simulink library "TestSeq_slave_lib"  (Simulink 8.1)
settings: Solver=ode45  StartTime=0.0  StopTime=10.0  RelTol=1e-3
undefined symbols (not defined in the file): DiscIntNeverNeededParam, Ts
libraries: simulink x24, simulink_extras x1
settings Model: Creator=ch24070  LastModifiedBy=pkoralew

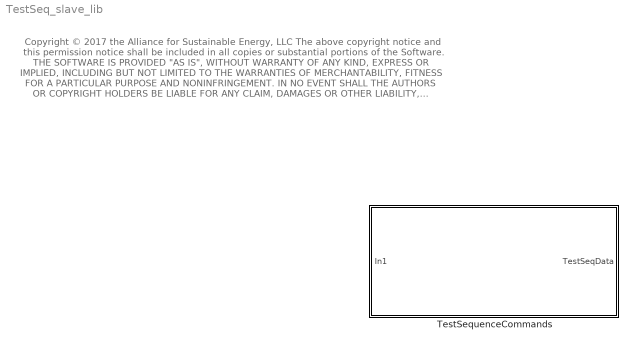
== system TestSeq_slave_lib ==
  note: Copyright © 2017 the Alliance for Sustainable Energy, LLC
      |
      | The above copyright notice and this permission notice shall be included in all copies or substantial portions of the Software.
      |
      | THE SOFTWARE IS PROVIDED "AS IS", WITHOUT WARRANTY OF ANY KIND, EXPRESS OR IMPLIED, INCLUDING
      | BUT NOT LIMITED TO THE WARRANTIES OF MERCHANTABILITY, FITNESS FOR A PARTICULAR PURPOSE AND
      | NONINFRINGEMENT. IN NO EVENT SHALL THE AUTHORS OR COPYRIGHT HOLDERS BE LIABLE FOR ANY CLAIM,
      |  DAMAGES OR OTHER LIABILITY, WHETHER IN AN ACTION OF CONTRACT, TORT OR OTHERWISE, ARISING FROM,
      | OUT OF OR IN CONNECTION WITH THE SOFTWARE OR THE USE OR OTHER DEALINGS IN THE SOFTWARE
  TestSequenceCommands : Subsystem

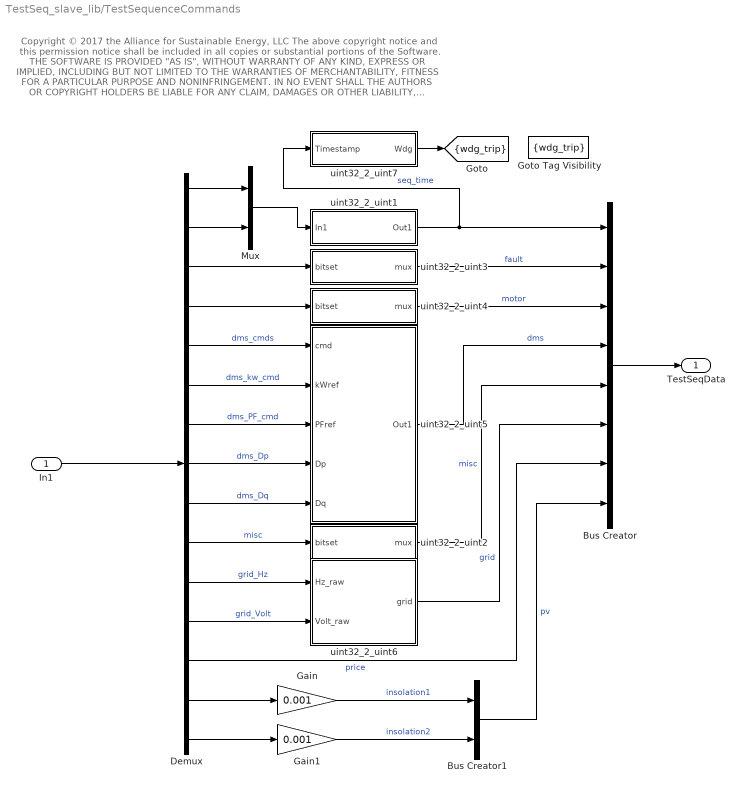
== system TestSeq_slave_lib/TestSequenceCommands ==
  note: Copyright © 2017 the Alliance for Sustainable Energy, LLC
      |
      | The above copyright notice and this permission notice shall be included in all copies or substantial portions of the Software.
      |
      | THE SOFTWARE IS PROVIDED "AS IS", WITHOUT WARRANTY OF ANY KIND, EXPRESS OR IMPLIED, INCLUDING
      | BUT NOT LIMITED TO THE WARRANTIES OF MERCHANTABILITY, FITNESS FOR A PARTICULAR PURPOSE AND
      | NONINFRINGEMENT. IN NO EVENT SHALL THE AUTHORS OR COPYRIGHT HOLDERS BE LIABLE FOR ANY CLAIM,
      |  DAMAGES OR OTHER LIABILITY, WHETHER IN AN ACTION OF CONTRACT, TORT OR OTHERWISE, ARISING FROM,
      | OUT OF OR IN CONNECTION WITH THE SOFTWARE OR THE USE OR OTHER DEALINGS IN THE SOFTWARE
  In1 : Inport
  Bus Creator : BusCreator  Inputs=8
  Bus Creator1 : BusCreator  Inputs=2
  Demux : Demux  Outputs=15
  Gain : Gain  Gain=0.001
  Gain1 : Gain  Gain=0.001
  Goto Tag Visibility : GotoTagVisibility  GotoTag=wdg_trip
  Mux : Mux  Inputs=2
  uint32_2_uint1 : Subsystem
      mask Display: disp('uint16_2_uint32');
  uint32_2_uint2 : Subsystem
  uint32_2_uint3 : Subsystem
  uint32_2_uint4 : Subsystem
  uint32_2_uint5 : Subsystem
  uint32_2_uint6 : Subsystem
  uint32_2_uint7 : Subsystem
      mask Display: disp('Watchdog\nT=2s');
  TestSeqData : Outport
  tag scope: wdg_trip=scoped
  wires:
  Gain1/1 -> Bus Creator1/2  "insolation2"
  Gain/1 -> Bus Creator1/1  "insolation1"
  Bus Creator1/1 -> Bus Creator/8  "pv"
  Demux/15 -> Gain1/1
  Demux/14 -> Gain/1
  uint32_2_uint6/1(grid) -> Bus Creator/6  "grid"
  uint32_2_uint7/1(Wdg) -> [wdg_trip]
  Demux/13 -> Bus Creator/7  "price"
  uint32_2_uint2/1(mux) -> Bus Creator/5  "misc"
  uint32_2_uint5/1(Out1) -> Bus Creator/4  "dms"
  uint32_2_uint4/1(mux) -> Bus Creator/3  "motor"
  uint32_2_uint3/1(mux) -> Bus Creator/2  "fault"
  Mux/1 -> uint32_2_uint1/1(In1)
  Demux/2 -> Mux/2
  Demux/1 -> Mux/1
  Demux/12 -> uint32_2_uint6/2(Volt_raw)  "grid_Volt"
  Demux/3 -> uint32_2_uint3/1(bitset)
  Demux/4 -> uint32_2_uint4/1(bitset)
  Demux/5 -> uint32_2_uint5/1(cmd)  "dms_cmds"
  Demux/6 -> uint32_2_uint5/2(kWref)  "dms_kw_cmd"
  Demux/7 -> uint32_2_uint5/3(PFref)  "dms_PF_cmd"
  Demux/8 -> uint32_2_uint5/4(Dp)  "dms_Dp"
  Demux/9 -> uint32_2_uint5/5(Dq)  "dms_Dq"
  Demux/10 -> uint32_2_uint2/1(bitset)  "misc"
  uint32_2_uint1/1(Out1) -> Bus Creator/1, uint32_2_uint7/1(Timestamp)  "seq_time"
  In1/1 -> Demux/1
  Demux/11 -> uint32_2_uint6/1(Hz_raw)  "grid_Hz"
  Bus Creator/1 -> TestSeqData/1

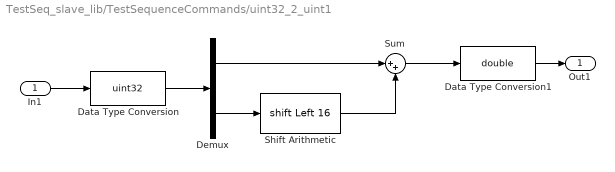
== system TestSeq_slave_lib/TestSequenceCommands/uint32_2_uint1 ==
  In1 : Inport
  Data Type Conversion : DataTypeConversion  OutDataTypeStr=uint32
  Data Type Conversion1 : DataTypeConversion  OutDataTypeStr=double
  Demux : Demux  Outputs=2
  Shift Arithmetic : ArithShift  BitShiftNumber=16  BitShiftDirection=Left
  Sum : Sum  Inputs=|++
  Out1 : Outport
  wires:
  Data Type Conversion/1 -> Demux/1
  Demux/1 -> Sum/1
  Demux/2 -> Shift Arithmetic/1
  Data Type Conversion1/1 -> Out1/1
  In1/1 -> Data Type Conversion/1
  Sum/1 -> Data Type Conversion1/1
  Shift Arithmetic/1 -> Sum/2

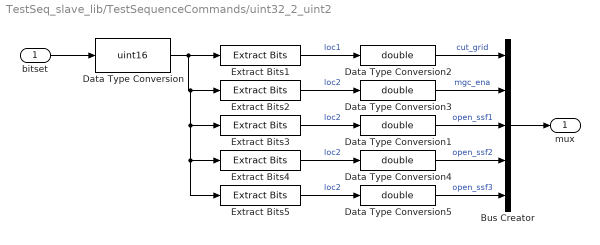
== system TestSeq_slave_lib/TestSequenceCommands/uint32_2_uint2 ==
  bitset : Inport
  Bus Creator : BusCreator  Inputs=5
  Data Type Conversion : DataTypeConversion  OutDataTypeStr=uint16
  Data Type Conversion{1..5} (5 alike) : DataTypeConversion  OutDataTypeStr=double
  Extract Bits1 : simulink/Logic and Bit Operations/Extract Bits  bitsToExtract=Range of bits  numBits=8  bitIdxRange=[0]  outScalingMode=Treat bit field as an integer
  Extract Bits2 : simulink/Logic and Bit Operations/Extract Bits  bitsToExtract=Range of bits  numBits=8  bitIdxRange=1  outScalingMode=Treat bit field as an integer
  Extract Bits3 : simulink/Logic and Bit Operations/Extract Bits  bitsToExtract=Range of bits  numBits=8  bitIdxRange=2  outScalingMode=Treat bit field as an integer
  Extract Bits4 : simulink/Logic and Bit Operations/Extract Bits  bitsToExtract=Range of bits  numBits=8  bitIdxRange=3  outScalingMode=Treat bit field as an integer
  Extract Bits5 : simulink/Logic and Bit Operations/Extract Bits  bitsToExtract=Range of bits  numBits=8  bitIdxRange=4  outScalingMode=Treat bit field as an integer
  mux : Outport
  wires:
  Extract Bits5/1 -> Data Type Conversion5/1  "loc2"
  Data Type Conversion5/1 -> Bus Creator/5  "open_ssf3"
  Extract Bits4/1 -> Data Type Conversion4/1  "loc2"
  Data Type Conversion4/1 -> Bus Creator/4  "open_ssf2"
  Data Type Conversion/1 -> Extract Bits1/1, Extract Bits2/1, Extract Bits3/1, Extract Bits4/1, Extract Bits5/1
  Extract Bits3/1 -> Data Type Conversion1/1  "loc2"
  Data Type Conversion1/1 -> Bus Creator/3  "open_ssf1"
  Extract Bits2/1 -> Data Type Conversion3/1  "loc2"
  Extract Bits1/1 -> Data Type Conversion2/1  "loc1"
  bitset/1 -> Data Type Conversion/1
  Bus Creator/1 -> mux/1
  Data Type Conversion2/1 -> Bus Creator/1  "cut_grid"
  Data Type Conversion3/1 -> Bus Creator/2  "mgc_ena"

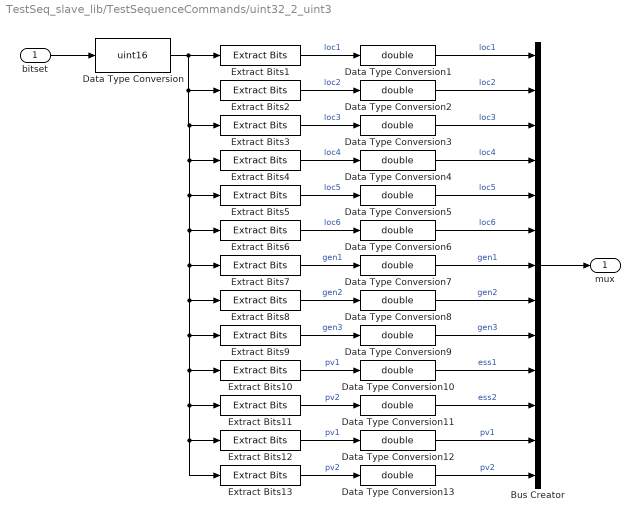
== system TestSeq_slave_lib/TestSequenceCommands/uint32_2_uint3 ==
  bitset : Inport
  Bus Creator : BusCreator  Inputs=13
  Data Type Conversion : DataTypeConversion  OutDataTypeStr=uint16
  Data Type Conversion{1..13} (13 alike) : DataTypeConversion  OutDataTypeStr=double
  Extract Bits1 : simulink/Logic and Bit Operations/Extract Bits  bitsToExtract=Range of bits  numBits=8  bitIdxRange=[0]  outScalingMode=Treat bit field as an integer
  Extract Bits10 : simulink/Logic and Bit Operations/Extract Bits  bitsToExtract=Range of bits  numBits=8  bitIdxRange=9  outScalingMode=Treat bit field as an integer
  Extract Bits11 : simulink/Logic and Bit Operations/Extract Bits  bitsToExtract=Range of bits  numBits=8  bitIdxRange=10  outScalingMode=Treat bit field as an integer
  Extract Bits12 : simulink/Logic and Bit Operations/Extract Bits  bitsToExtract=Range of bits  numBits=8  bitIdxRange=11  outScalingMode=Treat bit field as an integer
  Extract Bits13 : simulink/Logic and Bit Operations/Extract Bits  bitsToExtract=Range of bits  numBits=8  bitIdxRange=12  outScalingMode=Treat bit field as an integer
  Extract Bits2 : simulink/Logic and Bit Operations/Extract Bits  bitsToExtract=Range of bits  numBits=8  bitIdxRange=1  outScalingMode=Treat bit field as an integer
  Extract Bits3 : simulink/Logic and Bit Operations/Extract Bits  bitsToExtract=Range of bits  numBits=8  bitIdxRange=2  outScalingMode=Treat bit field as an integer
  Extract Bits4 : simulink/Logic and Bit Operations/Extract Bits  bitsToExtract=Range of bits  numBits=8  bitIdxRange=3  outScalingMode=Treat bit field as an integer
  Extract Bits5 : simulink/Logic and Bit Operations/Extract Bits  bitsToExtract=Range of bits  numBits=8  bitIdxRange=4  outScalingMode=Treat bit field as an integer
  Extract Bits6 : simulink/Logic and Bit Operations/Extract Bits  bitsToExtract=Range of bits  numBits=8  bitIdxRange=5  outScalingMode=Treat bit field as an integer
  Extract Bits7 : simulink/Logic and Bit Operations/Extract Bits  bitsToExtract=Range of bits  numBits=8  bitIdxRange=6  outScalingMode=Treat bit field as an integer
  Extract Bits8 : simulink/Logic and Bit Operations/Extract Bits  bitsToExtract=Range of bits  numBits=8  bitIdxRange=7  outScalingMode=Treat bit field as an integer
  Extract Bits9 : simulink/Logic and Bit Operations/Extract Bits  bitsToExtract=Range of bits  numBits=8  bitIdxRange=8  outScalingMode=Treat bit field as an integer
  mux : Outport
  wires:
  Extract Bits13/1 -> Data Type Conversion13/1  "pv2"
  Extract Bits12/1 -> Data Type Conversion12/1  "pv1"
  Data Type Conversion13/1 -> Bus Creator/13  "pv2"
  Data Type Conversion12/1 -> Bus Creator/12  "pv1"
  Data Type Conversion/1 -> Extract Bits2/1, Extract Bits3/1, Extract Bits13/1, Extract Bits12/1, Extract Bits11/1, Extract Bits10/1, Extract Bits9/1, Extract Bits8/1, Extract Bits7/1, Extract Bits6/1, Extract Bits5/1, Extract Bits4/1, Extract Bits1/1
  Extract Bits11/1 -> Data Type Conversion11/1  "pv2"
  Extract Bits10/1 -> Data Type Conversion10/1  "pv1"
  Extract Bits9/1 -> Data Type Conversion9/1  "gen3"
  Extract Bits8/1 -> Data Type Conversion8/1  "gen2"
  Extract Bits7/1 -> Data Type Conversion7/1  "gen1"
  Extract Bits6/1 -> Data Type Conversion6/1  "loc6"
  Extract Bits5/1 -> Data Type Conversion5/1  "loc5"
  Extract Bits4/1 -> Data Type Conversion4/1  "loc4"
  Extract Bits3/1 -> Data Type Conversion3/1  "loc3"
  Extract Bits2/1 -> Data Type Conversion2/1  "loc2"
  Extract Bits1/1 -> Data Type Conversion1/1  "loc1"
  Data Type Conversion11/1 -> Bus Creator/11  "ess2"
  Data Type Conversion10/1 -> Bus Creator/10  "ess1"
  Data Type Conversion9/1 -> Bus Creator/9  "gen3"
  Data Type Conversion8/1 -> Bus Creator/8  "gen2"
  Data Type Conversion7/1 -> Bus Creator/7  "gen1"
  Data Type Conversion6/1 -> Bus Creator/6  "loc6"
  Data Type Conversion5/1 -> Bus Creator/5  "loc5"
  Data Type Conversion4/1 -> Bus Creator/4  "loc4"
  Data Type Conversion3/1 -> Bus Creator/3  "loc3"
  Data Type Conversion2/1 -> Bus Creator/2  "loc2"
  Data Type Conversion1/1 -> Bus Creator/1  "loc1"
  Bus Creator/1 -> mux/1
  bitset/1 -> Data Type Conversion/1

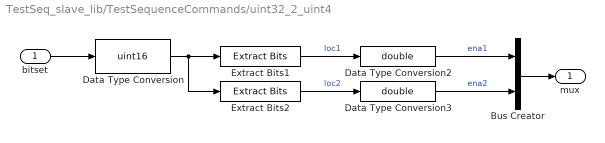
== system TestSeq_slave_lib/TestSequenceCommands/uint32_2_uint4 ==
  bitset : Inport
  Bus Creator : BusCreator  Inputs=2
  Data Type Conversion : DataTypeConversion  OutDataTypeStr=uint16
  Data Type Conversion2 : DataTypeConversion  OutDataTypeStr=double
  Data Type Conversion3 : DataTypeConversion  OutDataTypeStr=double
  Extract Bits1 : simulink/Logic and Bit Operations/Extract Bits  bitsToExtract=Range of bits  numBits=8  bitIdxRange=[0]  outScalingMode=Treat bit field as an integer
  Extract Bits2 : simulink/Logic and Bit Operations/Extract Bits  bitsToExtract=Range of bits  numBits=8  bitIdxRange=1  outScalingMode=Treat bit field as an integer
  mux : Outport
  wires:
  Extract Bits2/1 -> Data Type Conversion3/1  "loc2"
  Extract Bits1/1 -> Data Type Conversion2/1  "loc1"
  Data Type Conversion2/1 -> Bus Creator/1  "ena1"
  Data Type Conversion3/1 -> Bus Creator/2  "ena2"
  bitset/1 -> Data Type Conversion/1
  Bus Creator/1 -> mux/1
  Data Type Conversion/1 -> Extract Bits1/1, Extract Bits2/1

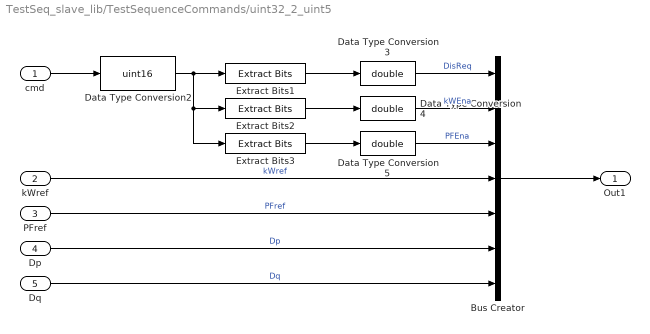
== system TestSeq_slave_lib/TestSequenceCommands/uint32_2_uint5 ==
  cmd : Inport
  kWref : Inport  Port=2
  PFref : Inport  Port=3
  Dp : Inport  Port=4
  Dq : Inport  Port=5
  Bus Creator : BusCreator  Inputs=7
  Data Type Conversion2 : DataTypeConversion  OutDataTypeStr=uint16
  Data Type Conversion3 : DataTypeConversion  OutDataTypeStr=double
  Data Type Conversion4 : DataTypeConversion  OutDataTypeStr=double
  Data Type Conversion5 : DataTypeConversion  OutDataTypeStr=double
  Extract Bits1 : simulink/Logic and Bit Operations/Extract Bits  bitsToExtract=Range of bits  numBits=8  bitIdxRange=[0]  outScalingMode=Treat bit field as an integer
  Extract Bits2 : simulink/Logic and Bit Operations/Extract Bits  bitsToExtract=Range of bits  numBits=8  bitIdxRange=1  outScalingMode=Treat bit field as an integer
  Extract Bits3 : simulink/Logic and Bit Operations/Extract Bits  bitsToExtract=Range of bits  numBits=8  bitIdxRange=2  outScalingMode=Treat bit field as an integer
  Out1 : Outport
  wires:
  Data Type Conversion5/1 -> Bus Creator/3  "PFEna"
  Data Type Conversion4/1 -> Bus Creator/2  "kWEna"
  Data Type Conversion3/1 -> Bus Creator/1  "DisReq"
  Dq/1 -> Bus Creator/7  "Dq"
  Dp/1 -> Bus Creator/6  "Dp"
  PFref/1 -> Bus Creator/5  "PFref"
  kWref/1 -> Bus Creator/4  "kWref"
  Data Type Conversion2/1 -> Extract Bits1/1, Extract Bits3/1, Extract Bits2/1
  Extract Bits3/1 -> Data Type Conversion5/1
  Extract Bits2/1 -> Data Type Conversion4/1
  Extract Bits1/1 -> Data Type Conversion3/1
  cmd/1 -> Data Type Conversion2/1
  Bus Creator/1 -> Out1/1

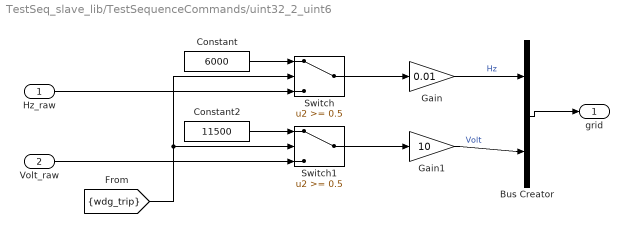
== system TestSeq_slave_lib/TestSequenceCommands/uint32_2_uint6 ==
  Hz_raw : Inport
  Volt_raw : Inport  Port=2
  Bus Creator : BusCreator  Inputs=2
  Constant : Constant  Value=6000
  Constant2 : Constant  Value=11500
  Gain : Gain  Gain=0.01
  Gain1 : Gain  Gain=10
  Switch : Switch  Threshold=0.5
  Switch1 : Switch  Threshold=0.5
  grid : Outport
  wires:
  Gain1/1 -> Bus Creator/2  "Volt"
  Gain/1 -> Bus Creator/1  "Hz"
  Switch1/1 -> Gain1/1
  Switch/1 -> Gain/1
  Constant2/1 -> Switch1/1
  Constant/1 -> Switch/1
  Volt_raw/1 -> Switch1/3
  Hz_raw/1 -> Switch/3
  [wdg_trip] -> Switch1/2, Switch/2
  Bus Creator/1 -> grid/1

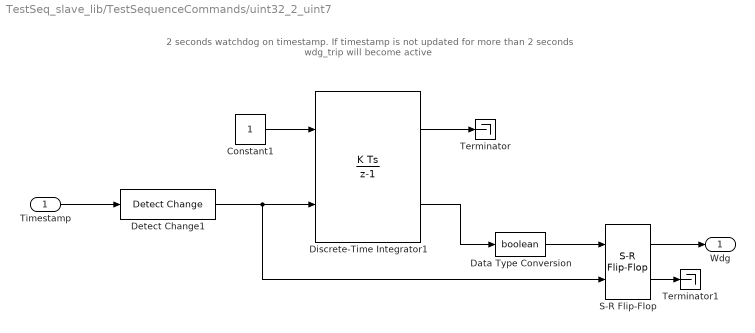
== system TestSeq_slave_lib/TestSequenceCommands/uint32_2_uint7 ==
  note: 2 seconds watchdog on timestamp.
      |  If timestamp is not updated for more than 2 seconds wdg_trip will become active
  Timestamp : Inport
  Constant1 : Constant
  Data Type Conversion : DataTypeConversion  OutDataTypeStr=boolean
  Detect Change1 : simulink/Logic and Bit Operations/Detect Change  vinit=0  InputProcessing=Inherited  OutDataTypeStr=boolean
  Discrete-Time Integrator1 : DiscreteIntegrator  ExternalReset=level  SampleTime=Ts  LimitOutput=on  UpperSaturationLimit=2  ShowSaturationPort=on  ICPrevOutput=DiscIntNeverNeededParam  ICPrevScaledInput=DiscIntNeverNeededParam
  S-R Flip-Flop : simulink_extras/Flip Flops/S-R Flip-Flop  initial_condition=1
  Terminator : Terminator
  Terminator1 : Terminator
  Wdg : Outport
  wires:
  S-R Flip-Flop/2 -> Terminator1/1
  S-R Flip-Flop/1 -> Wdg/1
  Discrete-Time Integrator1/1 -> Terminator/1
  Data Type Conversion/1 -> S-R Flip-Flop/1
  Constant1/1 -> Discrete-Time Integrator1/1
  Detect Change1/1 -> Discrete-Time Integrator1/2, S-R Flip-Flop/2
  Timestamp/1 -> Detect Change1/1
  Discrete-Time Integrator1/2 -> Data Type Conversion/1
